simulink subsystem "OES_Valve"  (R2023a)
settings: Solver=VariableStepAuto  StartTime=0.0  StopTime=10.0  RelTol=1e-3
undefined symbols (not defined in the file): SENS_STATUS
libraries: simulink x1
settings Model: Creator=michael.roesch  LastModifiedBy=michael.roesch

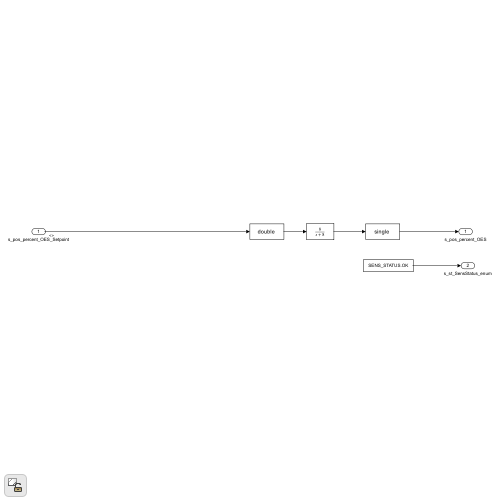
[thumbnail: Simulink's stored preview of the top-level diagram]
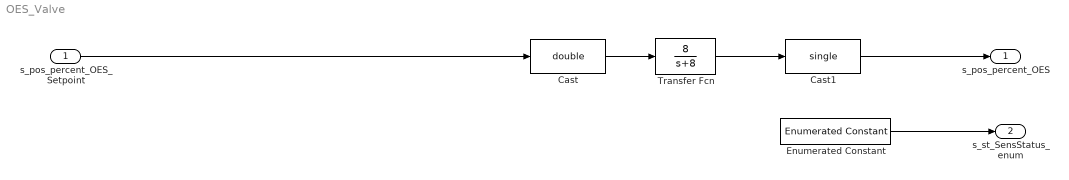
== system OES_Valve ==
  s_pos_percent_OES_Setpoint : Inport
  Cast : DataTypeConversion  OutDataTypeStr=double  SaturateOnIntegerOverflow=off  RndMeth=Floor
  Cast1 : DataTypeConversion  OutDataTypeStr=single  SaturateOnIntegerOverflow=off  RndMeth=Floor
  Enumerated Constant : simulink/Sources/Enumerated Constant  OutDataTypeStr=Enum: SENS_STATUS  Value=SENS_STATUS.OK  SampleTime=inf
  Transfer Fcn : TransferFcn  Numerator=[8]  Denominator=[1 8]
  s_pos_percent_OES : Outport
  s_st_SensStatus_enum : Outport  Port=2
  wires:
  Cast/1 -> Transfer Fcn/1
  Enumerated Constant/1 -> s_st_SensStatus_enum/1
  Transfer Fcn/1 -> Cast1/1
  s_pos_percent_OES_Setpoint/1 -> Cast/1
  Cast1/1 -> s_pos_percent_OES/1
